simulink library "ElectricalElements"  (R2019b)
settings: Solver=VariableStepAuto  StartTime=0.0  StopTime=10.0  RelTol=1e-3
undefined symbols (not defined in the file or in its folder): MaxOpVolt, MinOpVolt, R
libraries: fl_lib x17, nesl_utility x11, simulink x5, $bdroot x2
settings Model: Creator=alfon  LastModifiedBy=Alfonso
settings SFSimCC: CustomCodeUndefinedFunction=UseInterfaceOnly

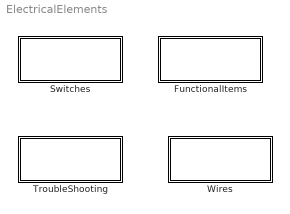
== system ElectricalElements ==
  FunctionalItems : Subsystem
  Switches : Subsystem
  TroubleShooting : Subsystem
  Wires : Subsystem

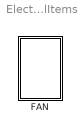
== system ElectricalElements/FunctionalItems ==
  FAN : Subsystem  mask{FanStatusTag=FAN1State, GotoTag=FAN1Fail, FANNumber=1, FanEnerTag=FAN1Energized}
      mask prompts: FanStatusTag "Fan Status Tag:"; GotoTag "Simulink:blkprm_prompts:FromGotoTag"; FANNumber "Fan Number:"; FanEnerTag "Fan Energized Tag:"
      settings: AttributesFormatString=FAN%<FANNumber>
      mask TypeOptions FanStatusTag: FANStatusTag/GotoTag
      mask TypeOptions GotoTag: FANFailTag/GotoTag
      mask TypeOptions FanEnerTag: FANEnergizedTag/GotoTag
      mask DialogControl GotoTag Prompt: Goto tag:

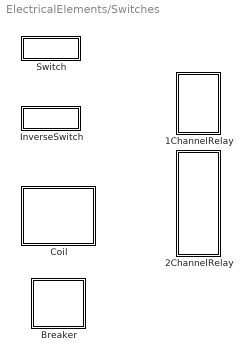
== system ElectricalElements/Switches ==
  1ChannelRelay : Subsystem  mask{R=100, MinOpVolt=32, MaxOpVolt=22, RelayStateTag=A, RelayFailModeTag=A}
      mask prompts: R "Relay Resistance:"; MinOpVolt "Max. Operation Voltage:"; MaxOpVolt "Min. Operation Voltage:"; RelayStateTag "Relay State Tag:"; RelayFailModeTag "Relay Fail Mode Tag:"
      mask TypeOptions R: Coil/R
      mask TypeOptions MinOpVolt: Coil/MinOpVolt
      mask TypeOptions MaxOpVolt: Coil/MaxOpVolt
      mask TypeOptions RelayStateTag: Coil/RelayStateTag
      mask TypeOptions RelayFailModeTag: Coil/RelayFailModeTag
  2ChannelRelay : Subsystem  mask{R=100, MinOpVolt=32, MaxOpVolt=22, RelayStateTag=A, RelayFailModeTag=A}
      mask prompts: R "Relay Resistance:"; MinOpVolt "Max. Operation Voltage:"; MaxOpVolt "Min. Operation Voltage:"; RelayStateTag "Relay State Tag:"; RelayFailModeTag "Relay Fail Mode Tag:"
      mask TypeOptions R: Coil/R
      mask TypeOptions MinOpVolt: Coil/MinOpVolt
      mask TypeOptions MaxOpVolt: Coil/MaxOpVolt
      mask TypeOptions RelayStateTag: Coil/RelayStateTag
      mask TypeOptions RelayFailModeTag: Coil/RelayFailModeTag
  Breaker : Subsystem  mask{GotoTag=BreakerCommand}
      mask prompts: GotoTag "Breaker Command Tag:"
      mask TypeOptions GotoTag: BreakerCommandTag/GotoTag
  Coil : Subsystem  mask{R=R, MinOpVolt=MinOpVolt, MaxOpVolt=MaxOpVolt, RelayStateTag=A, RelayFailModeTag=A}
      mask prompts: R "Relay Resistance:"; MinOpVolt "Max. Operation Voltage:"; MaxOpVolt "Min. Operation Voltage:"; RelayStateTag "Relay State Tag:"; RelayFailModeTag "Relay Fail Mode Tag:"
      mask TypeOptions R: Resistor/R
      mask TypeOptions MinOpVolt:
      | Compare
      | To Constant/const
      mask TypeOptions MaxOpVolt:
      | Compare
      | To Constant1/const
      mask TypeOptions RelayStateTag: RelayState/GotoTag
      mask TypeOptions RelayFailModeTag: RelayFailMode/GotoTag
  InverseSwitch : Subsystem  mask{SwitchTag=A}
      mask prompts: SwitchTag "Switch Control Tag:"
      settings: AttributesFormatString=Inverse %<SwitchTag>
      mask TypeOptions SwitchTag: SwitchControlTag/GotoTag
  Switch : Subsystem  mask{SwitchTag=A}
      mask prompts: SwitchTag "Switch Control Tag:"
      settings: AttributesFormatString=%<SwitchTag>
      mask TypeOptions SwitchTag: SwitchControlTag/GotoTag

== system ElectricalElements/TroubleShooting ==
  CurrentSensor : Subsystem

== system ElectricalElements/Wires ==
  Wire : Subsystem  mask{ResistanceTag=WireResistor, CurrentTag=WireCurrent, FailTag=WireFail}
      mask prompts: ResistanceTag "Resistance Tag:"; CurrentTag "Current Measurement Tag:"; FailTag "Wire Fail Tag:"
      settings: MoveFcn=|
      | WireNumeration(gcbh)
      | set_param(gcbh,'ResistanceTag',strcat(get_param(gcbh,'Name'),'Resistor'))
      | set_param(gcbh,'CurrentTag',strcat(get_param(gcbh,'Name'),'Current'))
      | set_param(gcbh,'FailTag',strcat(get_param(gcbh,'Name'),'Fail'))
      mask TypeOptions ResistanceTag: ResistanceTag/GotoTag
      mask TypeOptions CurrentTag: CurrentMeasurementTag/GotoTag
      mask TypeOptions FailTag: WireFailTag/GotoTag

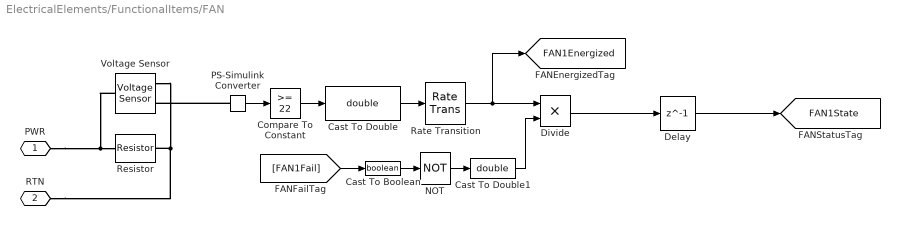
== system ElectricalElements/FunctionalItems/FAN ==
  Cast To Boolean : DataTypeConversion  OutDataTypeStr=boolean
  Cast To Double : DataTypeConversion  OutDataTypeStr=double
  Cast To Double1 : DataTypeConversion  OutDataTypeStr=double
  Compare To Constant : simulink/Logic and Bit Operations/Compare To Constant  relop=>=  const=22  OutDataTypeStr=boolean
  Delay : Delay  DelayLength=1  InitialCondition=0
  Divide : Product  Inputs=**
  NOT : Logic  Operator=NOT  IconShape=distinctive  AllPortsSameDT=off  OutDataTypeStr=boolean
  PS-Simulink Converter : nesl_utility/PS-Simulink Converter  PhysicalDomain=network_engine_domain  SubClassName=ps_output  LeftPortType=input  RightPortType=output  PseudoPeriodic=off  Frequencies=[]  Unit=1  AffineConversion=off
  Rate Transition : RateTransition
  Resistor : fl_lib/Electrical/Electrical Elements/Resistor  R=100 Ohm  i_specify=off  i_priority=None  i=0 A  i_nominal_specify=off  i_nominal_unit=A  i_nominal_value=1  v_specify=off  v_priority=None  v=0 V  v_nominal_specify=off  v_nominal_unit=V  v_nominal_value=1
  Voltage Sensor : fl_lib/Electrical/Electrical Sensors/Voltage Sensor
  PWR : PMIOPort  Side=Left
  RTN : PMIOPort  Port=2  Side=Left
  tag scope: FAN1Energized=global, FAN1State=global
  wires:
  PS-Simulink Converter/1 -> Compare To Constant/1
  Compare To Constant/1 -> Cast To Double/1
  Cast To Double/1 -> Rate Transition/1
  Divide/1 -> Delay/1
  [FAN1Fail] -> Cast To Boolean/1
  NOT/1 -> Cast To Double1/1
  Cast To Double1/1 -> Divide/2
  Delay/1 -> [FAN1State]
  Cast To Boolean/1 -> NOT/1
  Rate Transition/1 -> [FAN1Energized], Divide/1
  connections:
  Resistor/LConn1 -- Voltage Sensor/LConn1 -- PWR/RConn1
  Resistor/RConn1 -- Voltage Sensor/RConn2 -- RTN/RConn1
  PS-Simulink Converter/LConn1 -- Voltage Sensor/RConn1

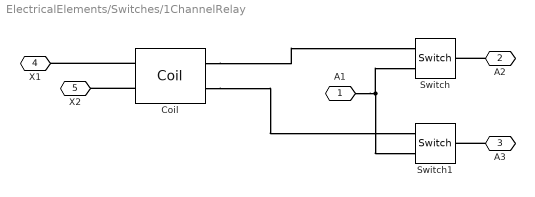
== system ElectricalElements/Switches/1ChannelRelay ==
  Coil : $bdroot/Switches/Coil  R=R  MinOpVolt=MinOpVolt  MaxOpVolt=MaxOpVolt  RelayStateTag=A  RelayFailModeTag=A
  Switch : fl_lib/Electrical/Electrical Elements/Switch  R_closed=0.01 Ohm  G_open=1e-8 1/Ohm  Threshold=0.5  i_specify=off  i_priority=None  i=0 A  i_nominal_specify=off  i_nominal_unit=A  i_nominal_value=1  v_specify=off  v_priority=None  v=0 V  v_nominal_specify=off  v_nominal_unit=V  v_nominal_value=1
      settings: SourceProductName=Simscape
  Switch1 : fl_lib/Electrical/Electrical Elements/Switch  R_closed=0.01 Ohm  G_open=1e-8 1/Ohm  Threshold=0.5  i_specify=off  i_priority=None  i=0 A  i_nominal_specify=off  i_nominal_unit=A  i_nominal_value=1  v_specify=off  v_priority=None  v=0 V  v_nominal_specify=off  v_nominal_unit=V  v_nominal_value=1
      settings: SourceProductName=Simscape
  A1 : PMIOPort  Side=Left
  A2 : PMIOPort  Port=2  Side=Right
  A3 : PMIOPort  Port=3  Side=Right
  X1 : PMIOPort  Port=4  Side=Left
  X2 : PMIOPort  Port=5  Side=Right
  connections:
  Coil/LConn2 -- X2/RConn1
  A1/RConn1 -- Switch1/RConn2 -- Switch/RConn2
  Coil/LConn1 -- X1/RConn1
  A2/RConn1 -- Switch/LConn1
  A3/RConn1 -- Switch1/LConn1
  Coil/RConn2 -- Switch1/RConn1
  Coil/RConn1 -- Switch/RConn1

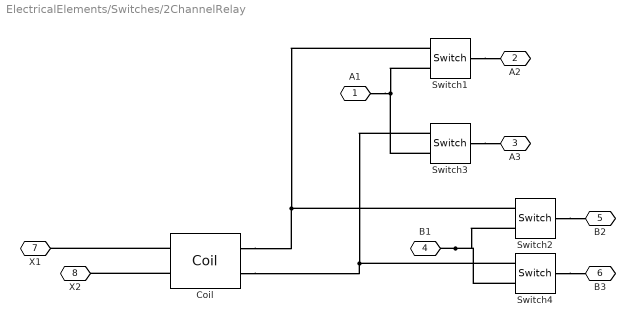
== system ElectricalElements/Switches/2ChannelRelay ==
  Coil : $bdroot/Switches/Coil  R=R  MinOpVolt=MinOpVolt  MaxOpVolt=MaxOpVolt  RelayStateTag=A  RelayFailModeTag=A
  Switch{1..4} (4 alike) : fl_lib/Electrical/Electrical Elements/Switch  R_closed=0.01 Ohm  G_open=1e-8 1/Ohm  Threshold=0.5  i_specify=off  i_priority=None  i=0 A  i_nominal_specify=off  i_nominal_unit=A  i_nominal_value=1  v_specify=off  v_priority=None  v=0 V  v_nominal_specify=off  v_nominal_unit=V  v_nominal_value=1
      settings: SourceProductName=Simscape
  A1 : PMIOPort  Side=Left
  A2 : PMIOPort  Port=2  Side=Right
  A3 : PMIOPort  Port=3  Side=Right
  B1 : PMIOPort  Port=4  Side=Left
  B2 : PMIOPort  Port=5  Side=Right
  B3 : PMIOPort  Port=6  Side=Right
  X1 : PMIOPort  Port=7  Side=Left
  X2 : PMIOPort  Port=8  Side=Right
  connections:
  Switch1/RConn1 -- Coil/RConn1 -- Switch2/RConn1
  Switch3/RConn1 -- Coil/RConn2 -- Switch4/RConn1
  Switch3/LConn1 -- A3/RConn1
  Switch1/LConn1 -- A2/RConn1
  Coil/LConn1 -- X1/RConn1
  A1/RConn1 -- Switch1/RConn2 -- Switch3/RConn2
  Coil/LConn2 -- X2/RConn1
  Switch4/LConn1 -- B3/RConn1
  B1/RConn1 -- Switch2/RConn2 -- Switch4/RConn2
  Switch2/LConn1 -- B2/RConn1

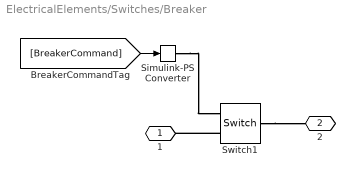
== system ElectricalElements/Switches/Breaker ==
  Simulink-PS Converter : nesl_utility/Simulink-PS Converter  PhysicalDomain=network_engine_domain  SubClassName=ps_input  LeftPortType=input  RightPortType=output  PseudoPeriodic=off  Frequencies=[]  NoiseDistribution=none  NoiseParameters=[]  Unit=1  AffineConversion=off  FilteringAndDerivatives=provide  SimscapeFilterOrder=1  InputFilterTimeConstant=0.001  UdotUserProvided=0
  Switch1 : fl_lib/Electrical/Electrical Elements/Switch  R_closed=0.01 Ohm  G_open=1e-8 1/Ohm  Threshold=0.5  i_specify=off  i_priority=None  i=0 A  i_nominal_specify=off  i_nominal_unit=A  i_nominal_value=1  v_specify=off  v_priority=None  v=0 V  v_nominal_specify=off  v_nominal_unit=V  v_nominal_value=1
      settings: SourceProductName=Simscape
  1 : PMIOPort  Side=Left
  2 : PMIOPort  Port=2  Side=Right
  wires:
  [BreakerCommand] -> Simulink-PS Converter/1
  connections:
  Switch1/LConn1 -- 2/RConn1
  Switch1/RConn2 -- 1/RConn1
  Simulink-PS Converter/RConn1 -- Switch1/RConn1

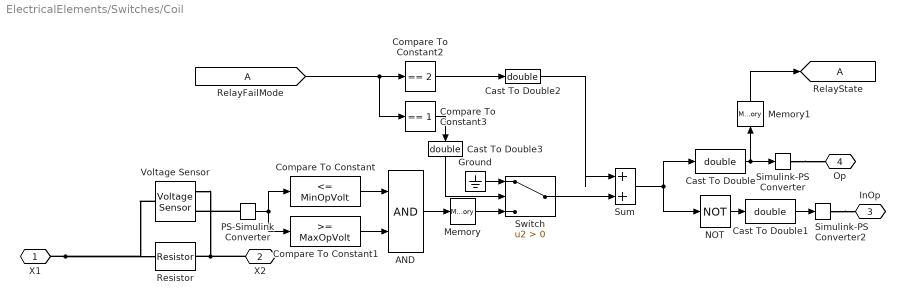
== system ElectricalElements/Switches/Coil ==
  AND : Logic  IconShape=distinctive  AllPortsSameDT=off  OutDataTypeStr=boolean
  Cast To Double{,1..3} (4 alike) : DataTypeConversion  OutDataTypeStr=double
  Compare To Constant : simulink/Logic and Bit Operations/Compare To Constant  relop=<=  const=MinOpVolt  OutDataTypeStr=boolean
  Compare To Constant1 : simulink/Logic and Bit Operations/Compare To Constant  relop=>=  const=MaxOpVolt  OutDataTypeStr=boolean
  Compare To Constant2 : simulink/Logic and Bit Operations/Compare To Constant  relop===  const=2  OutDataTypeStr=boolean
  Compare To Constant3 : simulink/Logic and Bit Operations/Compare To Constant  relop===  const=1  OutDataTypeStr=boolean
  Ground : Ground
  Memory : Memory
  Memory1 : Memory
  NOT : Logic  Operator=NOT  IconShape=distinctive  AllPortsSameDT=off  OutDataTypeStr=boolean
  PS-Simulink Converter : nesl_utility/PS-Simulink Converter  PhysicalDomain=network_engine_domain  SubClassName=ps_output  LeftPortType=input  RightPortType=output  PseudoPeriodic=off  Frequencies=[]  Unit=1  AffineConversion=off
  Resistor : fl_lib/Electrical/Electrical Elements/Resistor  R=R Ohm  i_specify=off  i_priority=None  i=0 A  i_nominal_specify=off  i_nominal_unit=A  i_nominal_value=1  v_specify=off  v_priority=None  v=0 V  v_nominal_specify=off  v_nominal_unit=V  v_nominal_value=1
  Simulink-PS Converter : nesl_utility/Simulink-PS Converter  PhysicalDomain=network_engine_domain  SubClassName=ps_input  LeftPortType=input  RightPortType=output  PseudoPeriodic=off  Frequencies=[]  NoiseDistribution=none  NoiseParameters=[]  Unit=1  AffineConversion=off  FilteringAndDerivatives=provide  SimscapeFilterOrder=1  InputFilterTimeConstant=0.001  UdotUserProvided=0
  Simulink-PS Converter2 : nesl_utility/Simulink-PS Converter  PhysicalDomain=network_engine_domain  SubClassName=ps_input  LeftPortType=input  RightPortType=output  PseudoPeriodic=off  Frequencies=[]  NoiseDistribution=none  NoiseParameters=[]  Unit=1  AffineConversion=off  FilteringAndDerivatives=provide  SimscapeFilterOrder=1  InputFilterTimeConstant=0.001  UdotUserProvided=0
  Sum : Sum  Inputs=|++
  Switch : Switch  Criteria=u2 > Threshold
  Voltage Sensor : fl_lib/Electrical/Electrical Sensors/Voltage Sensor
  X1 : PMIOPort  Side=Left
  X2 : PMIOPort  Port=2  Side=Left
  InOp : PMIOPort  Port=3  Side=Right
  Op : PMIOPort  Port=4  Side=Right
  tag scope: A=global
  wires:
  Cast To Double1/1 -> Simulink-PS Converter2/1
  NOT/1 -> Cast To Double1/1
  Compare To Constant/1 -> AND/1
  Cast To Double/1 -> Simulink-PS Converter/1, Memory1/1
  PS-Simulink Converter/1 -> Compare To Constant/1, Compare To Constant1/1
  Compare To Constant1/1 -> AND/2
  Sum/1 -> NOT/1, Cast To Double/1
  AND/1 -> Memory/1
  Switch/1 -> Sum/2
  [A] -> Compare To Constant3/1, Compare To Constant2/1
  Compare To Constant3/1 -> Cast To Double3/1
  Ground/1 -> Switch/1
  Compare To Constant2/1 -> Cast To Double2/1
  Cast To Double2/1 -> Sum/1
  Cast To Double3/1 -> Switch/2
  Memory/1 -> Switch/3
  Memory1/1 -> [A]
  connections:
  Simulink-PS Converter2/RConn1 -- InOp/RConn1
  X1/RConn1 -- Resistor/LConn1 -- Voltage Sensor/LConn1
  PS-Simulink Converter/LConn1 -- Voltage Sensor/RConn1
  X2/RConn1 -- Voltage Sensor/RConn2 -- Resistor/RConn1
  Simulink-PS Converter/RConn1 -- Op/RConn1

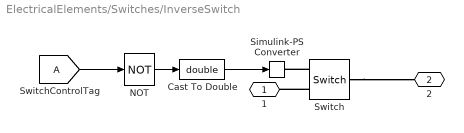
== system ElectricalElements/Switches/InverseSwitch ==
  Cast To Double : DataTypeConversion  OutDataTypeStr=double
  NOT : Logic  Operator=NOT  IconShape=distinctive  AllPortsSameDT=off  OutDataTypeStr=boolean
  Simulink-PS Converter : nesl_utility/Simulink-PS Converter  PhysicalDomain=network_engine_domain  SubClassName=ps_input  LeftPortType=input  RightPortType=output  PseudoPeriodic=off  Frequencies=[]  NoiseDistribution=none  NoiseParameters=[]  Unit=1  AffineConversion=off  FilteringAndDerivatives=provide  SimscapeFilterOrder=1  InputFilterTimeConstant=0.001  UdotUserProvided=0
  Switch : fl_lib/Electrical/Electrical Elements/Switch  R_closed=0.01 Ohm  G_open=1e-8 1/Ohm  Threshold=0.5  i_specify=off  i_priority=None  i=0 A  i_nominal_specify=off  i_nominal_unit=A  i_nominal_value=1  v_specify=off  v_priority=None  v=0 V  v_nominal_specify=off  v_nominal_unit=V  v_nominal_value=1
      settings: SourceProductName=Simscape
  1 : PMIOPort  Side=Left
  2 : PMIOPort  Port=2  Side=Right
  wires:
  [A] -> NOT/1
  NOT/1 -> Cast To Double/1
  Cast To Double/1 -> Simulink-PS Converter/1
  connections:
  Switch/RConn2 -- 1/RConn1
  Switch/LConn1 -- 2/RConn1
  Switch/RConn1 -- Simulink-PS Converter/RConn1

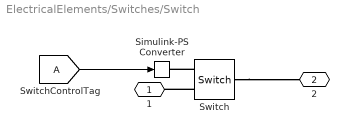
== system ElectricalElements/Switches/Switch ==
  Simulink-PS Converter : nesl_utility/Simulink-PS Converter  PhysicalDomain=network_engine_domain  SubClassName=ps_input  LeftPortType=input  RightPortType=output  PseudoPeriodic=off  Frequencies=[]  NoiseDistribution=none  NoiseParameters=[]  Unit=1  AffineConversion=off  FilteringAndDerivatives=provide  SimscapeFilterOrder=1  InputFilterTimeConstant=0.001  UdotUserProvided=0
  Switch : fl_lib/Electrical/Electrical Elements/Switch  R_closed=0.01 Ohm  G_open=1e-8 1/Ohm  Threshold=0.5  i_specify=off  i_priority=None  i=0 A  i_nominal_specify=off  i_nominal_unit=A  i_nominal_value=1  v_specify=off  v_priority=None  v=0 V  v_nominal_specify=off  v_nominal_unit=V  v_nominal_value=1
      settings: SourceProductName=Simscape
  1 : PMIOPort  Side=Left
  2 : PMIOPort  Port=2  Side=Right
  wires:
  [A] -> Simulink-PS Converter/1
  connections:
  Switch/RConn1 -- Simulink-PS Converter/RConn1
  Switch/LConn1 -- 2/RConn1
  Switch/RConn2 -- 1/RConn1

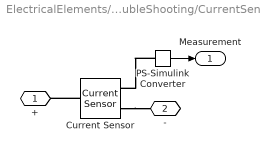
== system ElectricalElements/TroubleShooting/CurrentSensor ==
  Current Sensor : fl_lib/Electrical/Electrical Sensors/Current Sensor
  PS-Simulink Converter : nesl_utility/PS-Simulink Converter  PhysicalDomain=network_engine_domain  SubClassName=ps_output  LeftPortType=input  RightPortType=output  PseudoPeriodic=off  Frequencies=[]  Unit=1  AffineConversion=off
  + : PMIOPort  Side=Left
  - : PMIOPort  Port=2  Side=Right
  Measurement : Outport  VectorParamsAs1DForOutWhenUnconnected=off
  wires:
  PS-Simulink Converter/1 -> Measurement/1
  connections:
  Current Sensor/RConn2 -- -/RConn1
  PS-Simulink Converter/LConn1 -- Current Sensor/RConn1
  Current Sensor/LConn1 -- +/RConn1

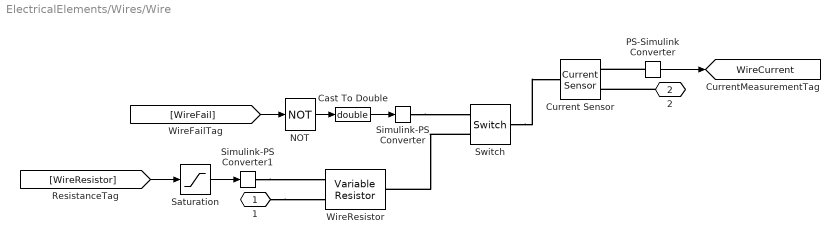
== system ElectricalElements/Wires/Wire ==
  Cast To Double : DataTypeConversion  OutDataTypeStr=double
  Current Sensor : fl_lib/Electrical/Electrical Sensors/Current Sensor
  NOT : Logic  Operator=NOT  IconShape=distinctive  AllPortsSameDT=off  OutDataTypeStr=boolean
  PS-Simulink Converter : nesl_utility/PS-Simulink Converter  PhysicalDomain=network_engine_domain  SubClassName=ps_output  LeftPortType=input  RightPortType=output  PseudoPeriodic=off  Frequencies=[]  Unit=1  AffineConversion=off
  Saturation : Saturate  UpperLimit=1e6  LowerLimit=1e-3
  Simulink-PS Converter : nesl_utility/Simulink-PS Converter  PhysicalDomain=network_engine_domain  SubClassName=ps_input  LeftPortType=input  RightPortType=output  PseudoPeriodic=off  Frequencies=[]  NoiseDistribution=none  NoiseParameters=[]  Unit=1  AffineConversion=off  FilteringAndDerivatives=provide  SimscapeFilterOrder=1  InputFilterTimeConstant=0.001  UdotUserProvided=0
  Simulink-PS Converter1 : nesl_utility/Simulink-PS Converter  PhysicalDomain=network_engine_domain  SubClassName=ps_input  LeftPortType=input  RightPortType=output  PseudoPeriodic=off  Frequencies=[]  NoiseDistribution=none  NoiseParameters=[]  Unit=1  AffineConversion=off  FilteringAndDerivatives=provide  SimscapeFilterOrder=1  InputFilterTimeConstant=0.001  UdotUserProvided=0
  Switch : fl_lib/Electrical/Electrical Elements/Switch  R_closed=0.01 Ohm  G_open=1e-8 1/Ohm  Threshold=0.5  i_specify=off  i_priority=None  i=0 A  i_nominal_specify=off  i_nominal_unit=A  i_nominal_value=1  v_specify=off  v_priority=None  v=0 V  v_nominal_specify=off  v_nominal_unit=V  v_nominal_value=1
      settings: SourceProductName=Simscape
  WireResistor : fl_lib/Electrical/Electrical Elements/Variable Resistor  Rmin=0 Ohm  i_specify=off  i_priority=None  i=0 A  i_nominal_specify=off  i_nominal_unit=A  i_nominal_value=1  v_specify=off  v_priority=None  v=0 V  v_nominal_specify=off  v_nominal_unit=V  v_nominal_value=1
  1 : PMIOPort  Side=Left
  2 : PMIOPort  Port=2  Side=Right
  tag scope: WireCurrent=global
  wires:
  [WireFail] -> NOT/1
  PS-Simulink Converter/1 -> [WireCurrent]
  [WireResistor] -> Saturation/1
  NOT/1 -> Cast To Double/1
  Cast To Double/1 -> Simulink-PS Converter/1
  Saturation/1 -> Simulink-PS Converter1/1
  connections:
  Simulink-PS Converter1/RConn1 -- WireResistor/LConn1
  2/RConn1 -- Current Sensor/RConn2
  Simulink-PS Converter/RConn1 -- Switch/RConn1
  Switch/LConn1 -- Current Sensor/LConn1
  1/RConn1 -- WireResistor/LConn2
  PS-Simulink Converter/LConn1 -- Current Sensor/RConn1
  Switch/RConn2 -- WireResistor/RConn1
